simulink model "sampleModel1972_4_sub"  (R2023a)
settings: Solver=VariableStepAuto  StartTime=0.0  StopTime=10.0  RelTol=1e-3
libraries: hdlsllib x3
settings Model: Creator=user1  LastModifiedBy=user1
settings OptimizationCC: BlockReduction=off  ConditionallyExecuteInputs=off

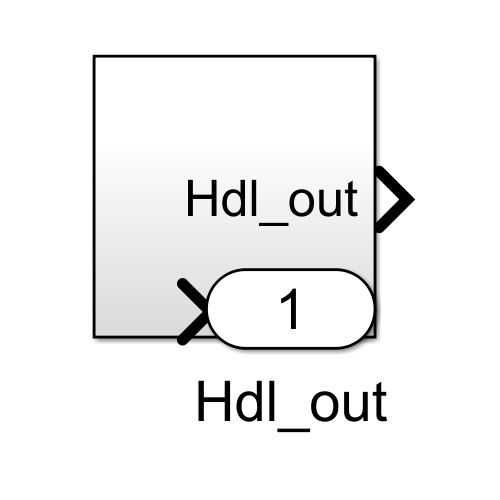
[thumbnail: Simulink's stored preview of the top-level diagram]
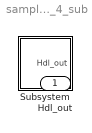
== system sampleModel1972_4_sub ==
  Subsystem : Subsystem
  Hdl_out : Outport  OutDataTypeStr=uint8

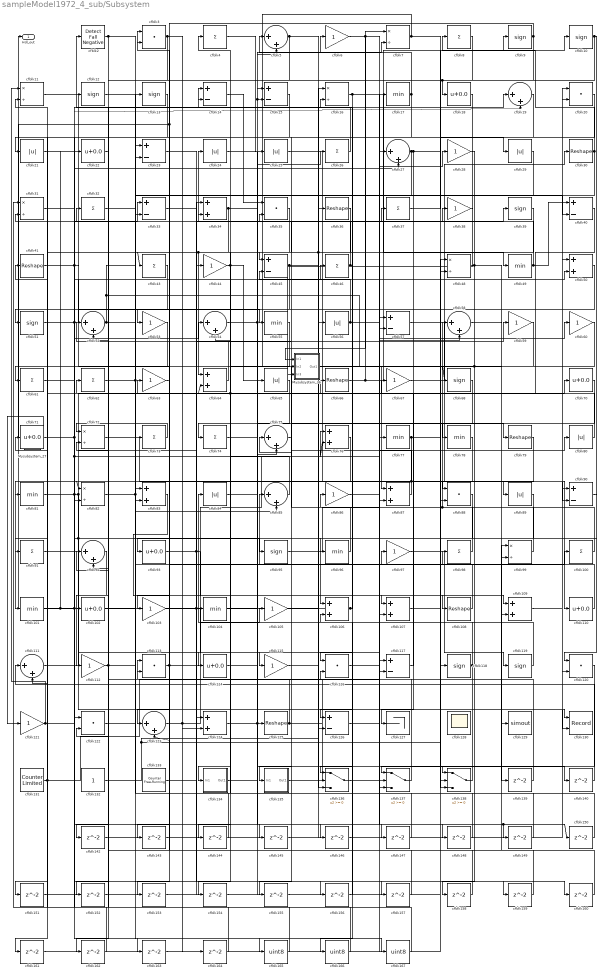
== system sampleModel1972_4_sub/Subsystem ==
  Mysubsystem_27 : Subsystem  TreatAsAtomicUnit=on  RTWFcnName=Mysubsystem_27
      settings: RTWFcnNameOpts=User specified  RTWFileNameOpts=Use function name
  Mysubsystem_36 : Subsystem  TreatAsAtomicUnit=on  RTWFcnName=Mysubsystem_36
      settings: RTWFcnNameOpts=User specified  RTWFileNameOpts=Use function name
  cfblk{9..10,12..13,39,51,68,95,118..119} (10 alike) : Signum
  cfblk{4,8,26,32,37,43,46,61..62,73..74,91,98,100} (14 alike) : Sum  Inputs=+  OutDataTypeStr=uint8
  cfblk{17,49,55,77..78,81,96,101,104} (9 alike) : MinMax  OutDataTypeStr=uint8
  cfblk{18,22,70..71,93,102,110,114} (8 alike) : Bias  Bias=0.0  SaturateOnIntegerOverflow=off
  cfblk{6,28,38,44,53,59..60,63,67,86,97,103,105,112,115,121} (16 alike) : Gain  OutDataTypeStr=uint8
  cfblk{34,50,64,76,83,87,106..107,109,124} (10 alike) : Sum  OutDataTypeStr=uint8
  cfblk{30,36,41,66,79,108,125} (7 alike) : Reshape
  cfblk{7,11,16,31,48,72,82,99} (8 alike) : Product  Inputs=*/  OutDataTypeStr=uint8  RndMeth=Zero  SaturateOnIntegerOverflow=on
  cfblk{5,19,27,52,54,58,75,85,92,111,123} (11 alike) : Sum  Inputs=|++  OutDataTypeStr=uint8
  cfblk{3,20,35,88,113,116,120,122} (8 alike) : DotProduct  OutDataTypeStr=uint8
  cfblk{14..15,23,33,40,45,57,90,117,126} (10 alike) : Sum  Inputs=+-  OutDataTypeStr=uint8
  cfblk127 : Terminator
  cfblk128 : Scope
      settings: Floating=on
  cfblk129 : ToWorkspace  VariableName=simout  SaveFormat=Timeseries  SampleTime=-1
  cfblk130 : Record  FileSettingsInternal="{\"entries\":[{\"content\":{\"excelSettings\":{\"content\":{},\"type\":\"Streamout.ExcelSettings\"}},\"type\":\"Streamout.FileSettingStorage\",\"uuid\":\"\"}],\"packageUris\":[\"http:\\/\\/schema.mathworks.com\\/mf0\\/streamout_blocks\\/R2020a\"],\"version\":\"1.0\"}"  Layout=[1 1]  SignalsInternal="{\"entries\":[{\"content\":{\"signals\":[{\"content\":{\"blockPath\":[],\"dimensions\":[1],\"domain\":\"\",\"lineColor\":\"#a2142f\",\"plots\":[1],\"port\":1,\"signalID\":56031,\"signalName\":\"cfblk91\"},\"type\":\"RecordBlkView.Signal\",\"uuid\":\"\"},{\"content\":{\"blockPath\":[],\"dimensions\":[1],\"domain\":\"\",\"lineColor\":\"#139fff\",\"plots\":[1],\"port\":2,\"signalID\":56034,\"signalName\":\"cfblk77\"},\"type\":\"RecordBlkView.Signal\",\"uuid\":\"\"}]},\"type\":\"RecordBlkView.InputSignals\",\"uuid\":\"\"}],\"packageUris\":[\"http:\\/\\/schema.mathworks.com\\/mf0\\/streamout_blocks\\/R2020a\"],\"version\":\"1.0\"}"  VisualizationBindings="{\"xyplotplugin\":{\"info\":[{\"series\":[{\"bindingParametersList\":[{\"parameter\":\"X-Axis\",\"signalID\":56031,\"signalName\":\"cfblk91\"},{\"parameter\":\"Y-Axis\",\"signalID\":56034,\"signalName\":\"cfblk77\"}],\"seriesID\":18770}],\"subplotID\":1}]}}"  CompatibilityTag=XY  st=-1
  cfblk131 : hdlsllib/Sources/Counter Limited  uplimit=7  tsamp=-1
  cfblk132 : Constant  OutDataTypeStr=uint8  SampleTime=-1
  cfblk133 : hdlsllib/Sources/Counter Free-Running  NumBits=16  tsamp=-1
  cfblk134 : Subsystem
      settings: LibrarySourceBlock=|
      | hdlsllib/Ports &
      | Subsystems/Subsystem
  cfblk135 : Subsystem
      settings: LibrarySourceBlock=|
      | hdlsllib/Ports &
      | Subsystems/Subsystem
  cfblk136 : Switch  OutDataTypeStr=uint8  SaturateOnIntegerOverflow=off  InputSameDT=off
  cfblk137 : Switch  OutDataTypeStr=uint8  SaturateOnIntegerOverflow=off  InputSameDT=off
  cfblk138 : Switch  OutDataTypeStr=uint8  SaturateOnIntegerOverflow=off  InputSameDT=off
  cfblk{139..140,142..164} (25 alike) : Delay  SampleTime=1
  cfblk165 : DataTypeConversion  OutDataTypeStr=uint8  SaturateOnIntegerOverflow=off  RndMeth=Floor
  cfblk166 : DataTypeConversion  OutDataTypeStr=uint8  SaturateOnIntegerOverflow=off  RndMeth=Floor
  cfblk167 : DataTypeConversion  OutDataTypeStr=uint8  SaturateOnIntegerOverflow=off  RndMeth=Floor
  cfblk2 : hdlsllib/Logic and Bit Operations/Detect Fall Negative  vinit=0  OutDataTypeStr=uint8
  cfblk{21,24..25,29,56,65,80,84,89} (9 alike) : Abs  OutDataTypeStr=uint8  SaturateOnIntegerOverflow=off
  Hdl_out : Outport  OutDataTypeStr=uint8
  wires:
  cfblk113/1 -> cfblk123/2, cfblk105/1
  cfblk17/1 -> cfblk82/2, cfblk5/1
  cfblk52/1 -> cfblk85/2, cfblk51/1
  cfblk67/1 -> cfblk30/1
  cfblk16/1 -> cfblk136/1, cfblk49/1
  cfblk40/1 -> cfblk62/1
  cfblk59/1 -> cfblk87/1
  cfblk10/1 -> cfblk126/2, cfblk93/1
  cfblk46/1 -> cfblk96/1, cfblk24/1
  cfblk14/1 -> cfblk35/1
  cfblk4/1 -> cfblk25/1
  cfblk9/1 -> cfblk138/3, cfblk61/1
  cfblk97/1 -> cfblk119/1
  cfblk66/1 -> cfblk7/1, cfblk9/1
  cfblk83/1 -> cfblk108/1
  cfblk88/1 -> cfblk106/1
  cfblk102/1 -> cfblk13/1
  cfblk70/1 -> cfblk116/1
  cfblk100/1 -> cfblk86/1
  cfblk82/1 -> cfblk159/1, cfblk76/1
  cfblk30/1 -> cfblk33/2, cfblk8/1
  cfblk120/1 -> cfblk137/1
  cfblk11/1 -> cfblk99/2
  cfblk96/1 -> cfblk75/1
  cfblk25/1 -> cfblk110/1
  cfblk118/1 -> cfblk104/1, cfblk113/1
  cfblk93/1 -> cfblk39/1, cfblk109/1
  cfblk20/1 -> cfblk45/1
  cfblk23/1 -> cfblk115/1
  cfblk134/1(Out1) -> cfblk75/2
  cfblk36/1 -> cfblk136/2, cfblk43/1
  cfblk131/1 -> cfblk71/1, cfblk57/1
  cfblk49/1 -> cfblk40/1, cfblk3/1
  cfblk95/1 -> cfblk77/1
  cfblk57/1 -> cfblk89/1
  cfblk119/1 -> cfblk84/1
  cfblk26/1 -> cfblk2/1
  cfblk34/1 -> cfblk91/1, cfblk7/2, cfblk15/2
  cfblk99/1 -> cfblk34/2
  cfblk123/1 -> cfblk124/2, cfblk57/2
  cfblk2/1 -> cfblk142/1, cfblk40/2
  cfblk98/1 -> cfblk52/1, cfblk58/1
  cfblk109/1 -> cfblk50/1
  cfblk21/1 -> cfblk109/2
  cfblk48/1 -> cfblk88/1, cfblk129/1
  cfblk87/1 -> cfblk82/1, cfblk31/2
  cfblk101/1 -> cfblk22/1, cfblk160/1, cfblk19/2
  cfblk13/1 -> cfblk21/1
  cfblk77/1 -> cfblk166/1, cfblk130/2
  cfblk6/1 -> cfblk148/1, Mysubsystem_36/1(In1)
  cfblk24/1 -> cfblk107/1
  cfblk117/1 -> cfblk67/1
  cfblk72/1 -> cfblk118/1
  cfblk27/1 -> cfblk136/3, cfblk90/2, cfblk127/1
  cfblk105/1 -> cfblk70/1
  cfblk112/1 -> cfblk152/1, cfblk97/1
  cfblk132/1 -> cfblk48/2, cfblk56/1
  cfblk65/1 -> cfblk134/1(In1)
  cfblk75/1 -> cfblk35/2
  cfblk35/1 -> cfblk153/1, cfblk64/1
  cfblk91/1 -> cfblk130/1
  cfblk61/1 -> cfblk54/1
  cfblk7/1 -> cfblk29/1, Mysubsystem_36/2(In2)
  cfblk63/1 -> cfblk103/1
  cfblk81/1 -> cfblk46/1, cfblk44/1, cfblk125/1, cfblk114/1
  cfblk74/1 -> cfblk79/1
  cfblk111/1 -> cfblk48/1
  cfblk51/1 -> cfblk163/1, cfblk20/2
  cfblk44/1 -> cfblk65/1, cfblk74/1
  cfblk121/1 -> cfblk11/1, cfblk76/2, cfblk19/1
  cfblk115/1 -> cfblk98/1
  cfblk12/1 -> cfblk73/1
  cfblk108/1 -> cfblk85/1
  cfblk73/1 -> cfblk72/1
  cfblk38/1 -> cfblk54/2
  cfblk138/1 -> cfblk14/1
  cfblk136/1 -> cfblk28/1
  cfblk106/1 -> Hdl_out/1, cfblk16/2
  cfblk80/1 -> cfblk41/1
  cfblk8/1 -> cfblk18/1, cfblk123/1, Mysubsystem_27/1(In1)
  cfblk85/1 -> cfblk64/2, cfblk4/1
  cfblk41/1 -> cfblk145/1, cfblk55/1
  cfblk137/1 -> cfblk72/2
  cfblk43/1 -> cfblk83/2
  cfblk84/1 -> cfblk6/1
  cfblk104/1 -> cfblk37/1
  cfblk76/1 -> cfblk101/1
  cfblk3/1 -> cfblk164/1, cfblk23/2
  cfblk56/1 -> cfblk58/2, cfblk45/2
  cfblk45/1 -> cfblk138/1, cfblk81/1
  cfblk135/1(Out1) -> cfblk17/1
  cfblk64/1 -> cfblk32/1
  cfblk107/1 -> cfblk100/1
  cfblk133/1 -> cfblk59/1
  cfblk92/1 -> cfblk112/1
  cfblk124/1 -> cfblk147/1, cfblk66/1
  cfblk15/1 -> cfblk111/2
  cfblk19/1 -> cfblk53/1
  cfblk126/1 -> cfblk38/1
  cfblk116/1 -> cfblk60/1
  cfblk54/1 -> cfblk146/1, cfblk26/1
  cfblk103/1 -> cfblk157/1, cfblk117/2
  cfblk86/1 -> cfblk80/1
  cfblk22/1 -> cfblk102/1
  cfblk90/1 -> cfblk120/1
  cfblk79/1 -> cfblk137/3
  cfblk125/1 -> cfblk12/1, cfblk87/2
  cfblk89/1 -> cfblk126/1
  cfblk5/1 -> cfblk92/2, cfblk36/1
  cfblk71/1 -> cfblk33/1, cfblk95/1
  cfblk110/1 -> cfblk63/1
  cfblk60/1 -> cfblk135/1(In1)
  cfblk31/1 -> cfblk27/2
  cfblk29/1 -> cfblk68/1, cfblk78/1
  cfblk37/1 -> cfblk10/1
  cfblk62/1 -> cfblk107/2, cfblk50/2
  cfblk58/1 -> cfblk139/1
  cfblk139/1 -> cfblk106/2
  cfblk114/1 -> cfblk140/1
  cfblk140/1 -> cfblk111/1
  cfblk142/1 -> cfblk16/1
  cfblk50/1 -> cfblk143/1
  cfblk143/1 -> cfblk20/1
  cfblk55/1 -> cfblk144/1
  cfblk144/1 -> cfblk83/1
  cfblk145/1 -> cfblk90/1
  cfblk146/1 -> cfblk120/2
  cfblk147/1 -> cfblk117/1
  cfblk148/1 -> cfblk113/2
  cfblk149/1 -> cfblk23/1
  cfblk150/1 -> cfblk14/2
  cfblk151/1 -> cfblk124/1
  cfblk152/1 -> cfblk138/2
  cfblk153/1 -> cfblk5/2
  cfblk78/1 -> cfblk154/1
  cfblk154/1 -> cfblk15/1
  cfblk68/1 -> cfblk155/1
  cfblk155/1 -> cfblk137/2
  cfblk33/1 -> cfblk156/1
  cfblk156/1 -> cfblk116/2
  cfblk157/1 -> cfblk52/2
  cfblk28/1 -> cfblk158/1
  cfblk158/1 -> cfblk34/1
  cfblk159/1 -> cfblk99/1
  cfblk160/1 -> cfblk3/2
  cfblk53/1 -> cfblk161/1
  cfblk161/1 -> cfblk27/1
  cfblk39/1 -> cfblk162/1
  cfblk162/1 -> cfblk31/1
  cfblk163/1 -> cfblk88/2
  cfblk164/1 -> cfblk11/2
  cfblk122/1 -> cfblk165/1
  cfblk165/1 -> cfblk92/1
  cfblk166/1 -> cfblk122/1
  cfblk32/1 -> cfblk167/1
  cfblk167/1 -> cfblk122/2
  Mysubsystem_27/1(Out1) -> cfblk121/1
  Mysubsystem_36/1(Out1) -> cfblk151/1, cfblk150/1, cfblk149/1
  cfblk18/1 -> Mysubsystem_36/3(In3)

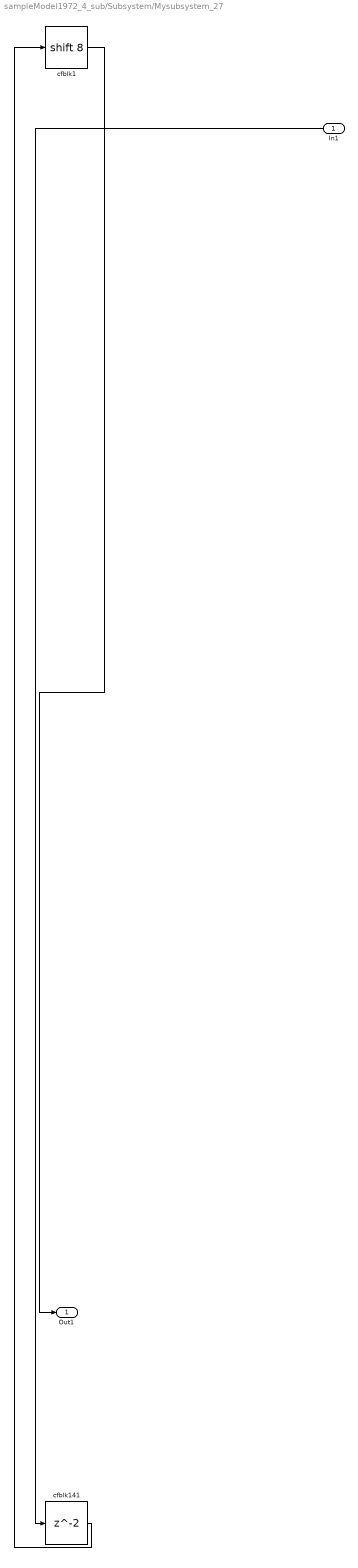
== system sampleModel1972_4_sub/Subsystem/Mysubsystem_27 ==
  In1 : Inport
  cfblk1 : ArithShift  BitShiftNumber=8
  cfblk141 : Delay  SampleTime=1
  Out1 : Outport
  wires:
  In1/1 -> cfblk141/1
  cfblk1/1 -> Out1/1
  cfblk141/1 -> cfblk1/1

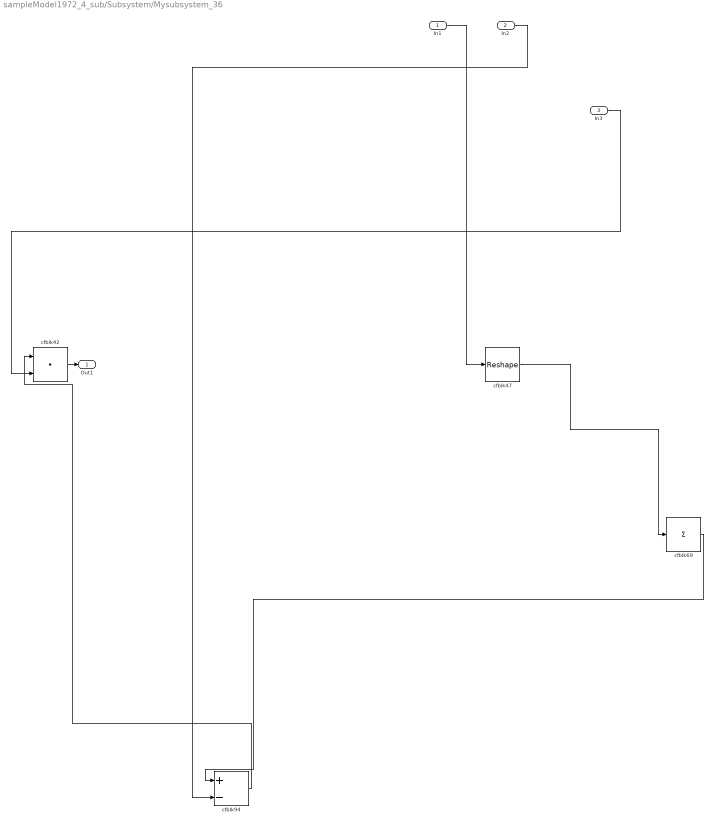
== system sampleModel1972_4_sub/Subsystem/Mysubsystem_36 ==
  In1 : Inport
  In2 : Inport  Port=2
  In3 : Inport  Port=3
  cfblk42 : DotProduct  OutDataTypeStr=Inherit: Inherit via internal rule
  cfblk47 : Reshape
  cfblk69 : Sum  Inputs=+
  cfblk94 : Sum  Inputs=+-
  Out1 : Outport
  wires:
  cfblk42/1 -> Out1/1
  In1/1 -> cfblk47/1
  cfblk69/1 -> cfblk94/1
  cfblk47/1 -> cfblk69/1
  In2/1 -> cfblk94/2
  cfblk94/1 -> cfblk42/1
  In3/1 -> cfblk42/2

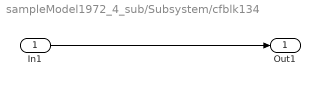
== system sampleModel1972_4_sub/Subsystem/cfblk134 ==
  In1 : Inport
  Out1 : Outport
  wires:
  In1/1 -> Out1/1

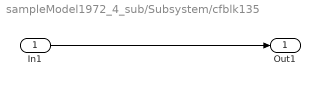
== system sampleModel1972_4_sub/Subsystem/cfblk135 ==
  In1 : Inport
  Out1 : Outport
  wires:
  In1/1 -> Out1/1
